simulink model "Q1_part4"  (R2019b)
settings: Solver=VariableStepAuto  StartTime=0.0  StopTime=10.0  RelTol=1e-3
settings Model: Creator=amirhosein  LastModifiedBy=amirhosein

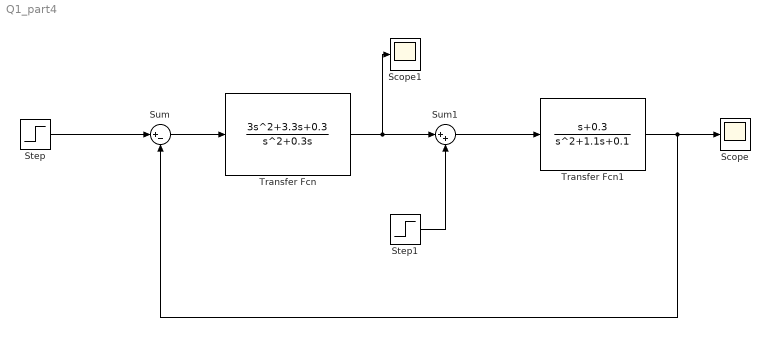
== system Q1_part4 ==
  Scope : Scope
  Scope1 : Scope
  Step : Step  Time=0  SampleTime=0
  Step1 : Step  Time=0  SampleTime=0
  Sum : Sum  Inputs=|+-
  Sum1 : Sum  Inputs=|++
  Transfer Fcn : TransferFcn  Numerator=[3 3.3 0.3]  Denominator=[1 0.3 0]
  Transfer Fcn1 : TransferFcn  Numerator=[1 0.3]  Denominator=[1 1.1 0.1]
  wires:
  Step/1 -> Sum/1
  Sum/1 -> Transfer Fcn/1
  Transfer Fcn/1 -> Scope1/1, Sum1/1
  Sum1/1 -> Transfer Fcn1/1
  Transfer Fcn1/1 -> Sum/2, Scope/1
  Step1/1 -> Sum1/2
